simulink model "unconnected_lines_2013a"  (R2013a)
settings: Solver=ode45  StartTime=0.0  StopTime=10.0  RelTol=1e-3
settings Model: Creator=ladmin  LastModifiedBy=ladmin
settings DebuggingCC: StateNameClashWarn=none

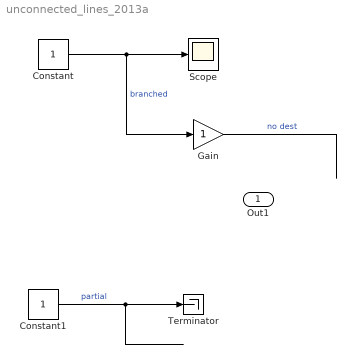
== system unconnected_lines_2013a ==
  Constant : Constant
  Constant1 : Constant
  Gain : Gain
  Scope : Scope
  Terminator : Terminator
  Out1 : Outport
  wires:
  Constant/1 -> Gain/1, Scope/1  "branched"
  Gain/1 -> ?  "no dest"
  ? -> Out1/1  "no source"
  ? -> ?  "free"
  Constant1/1 -> Terminator/1  "partial"
